simulink subsystem "Salida_Motores"  (R2024b)
settings: Solver=VariableStepAuto  StartTime=0.0  StopTime=10.0  RelTol=1e-3
libraries: arduinolib x6, simulink x2
settings Model: Creator=Chenfu  LastModifiedBy=lucia
settings OptimizationCC: ReuseModelBlockBuffer=off
settings RTWCC: GPUComputeCapability=3.5

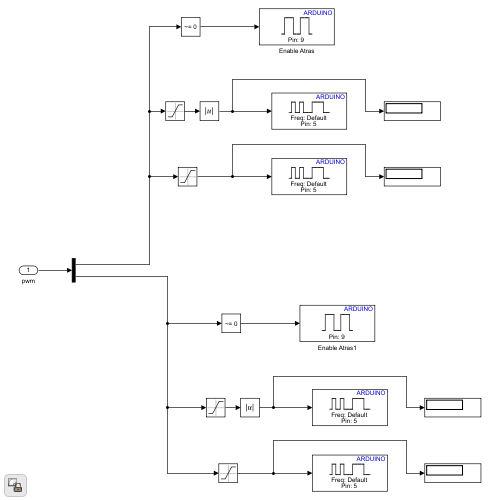
[thumbnail: Simulink's stored preview of the top-level diagram]
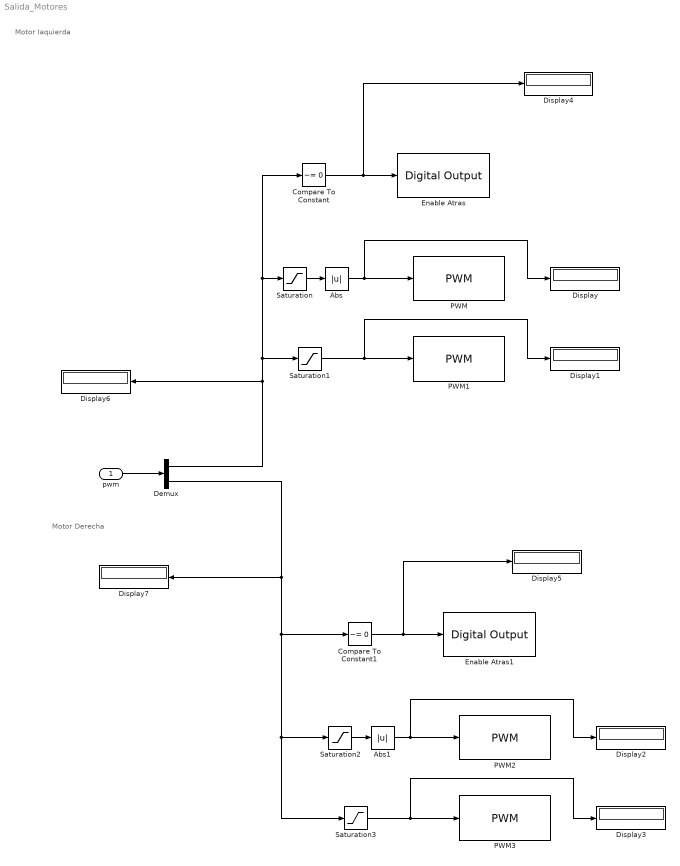
== system Salida_Motores ==
  note: Motor Derecha
  note: Motor Iaquierda
  pwm : Inport
  Abs : Abs  SaturateOnIntegerOverflow=off
  Abs1 : Abs  SaturateOnIntegerOverflow=off
  Compare To Constant : simulink/Logic and Bit Operations/Compare To Constant  relop=~=  const=0  OutDataTypeStr=boolean
  Compare To Constant1 : simulink/Logic and Bit Operations/Compare To Constant  relop=~=  const=0  OutDataTypeStr=boolean
  Demux : Demux  Outputs=2
  Display{,1..7} (8 alike) : Display
  Enable Atras : arduinolib/Digital Output  pinNumber=49  Direction=output  blockPlatform=arduino
  Enable Atras1 : arduinolib/Digital Output  pinNumber=48  Direction=output  blockPlatform=arduino
  PWM : arduinolib/PWM  pinNumber=3  frequencyType=Default  desiredFrequency=490.2  achievableFrequency=490.2
  PWM1 : arduinolib/PWM  pinNumber=4  frequencyType=Default  desiredFrequency=490.2  achievableFrequency=490.2
  PWM2 : arduinolib/PWM  pinNumber=2  frequencyType=Default  desiredFrequency=490.2  achievableFrequency=490.2
  PWM3 : arduinolib/PWM  pinNumber=5  frequencyType=Default  desiredFrequency=490.2  achievableFrequency=490.2
  Saturation : Saturate  UpperLimit=0  LowerLimit=-255
  Saturation1 : Saturate  UpperLimit=255  LowerLimit=0
  Saturation2 : Saturate  UpperLimit=0  LowerLimit=-255
  Saturation3 : Saturate  UpperLimit=255  LowerLimit=0
  wires:
  pwm/1 -> Demux/1
  Abs/1 -> Display/1, PWM/1
  Demux/1 -> Saturation/1, Compare To Constant/1, Saturation1/1, Display6/1
  Saturation/1 -> Abs/1
  Saturation1/1 -> PWM1/1, Display1/1
  Compare To Constant/1 -> Enable Atras/1, Display4/1
  Saturation3/1 -> PWM3/1, Display3/1
  Saturation2/1 -> Abs1/1
  Compare To Constant1/1 -> Enable Atras1/1, Display5/1
  Abs1/1 -> Display2/1, PWM2/1
  Demux/2 -> Display7/1, Saturation2/1, Saturation3/1, Compare To Constant1/1
